simulink library "scp"  (R2021b)
settings: Solver=VariableStepAuto  StartTime=0.0  StopTime=10.0  RelTol=1e-3
libraries: FVT_lib x1
settings Model: Creator=FVT23118  LastModifiedBy=FVT23010

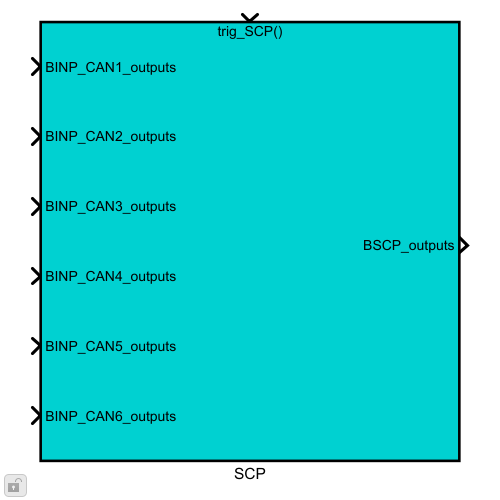
[thumbnail: Simulink's stored preview of the top-level diagram]
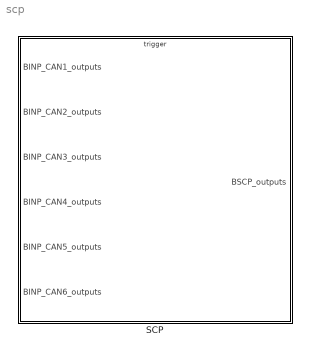
== system scp ==
  SCP : Subsystem

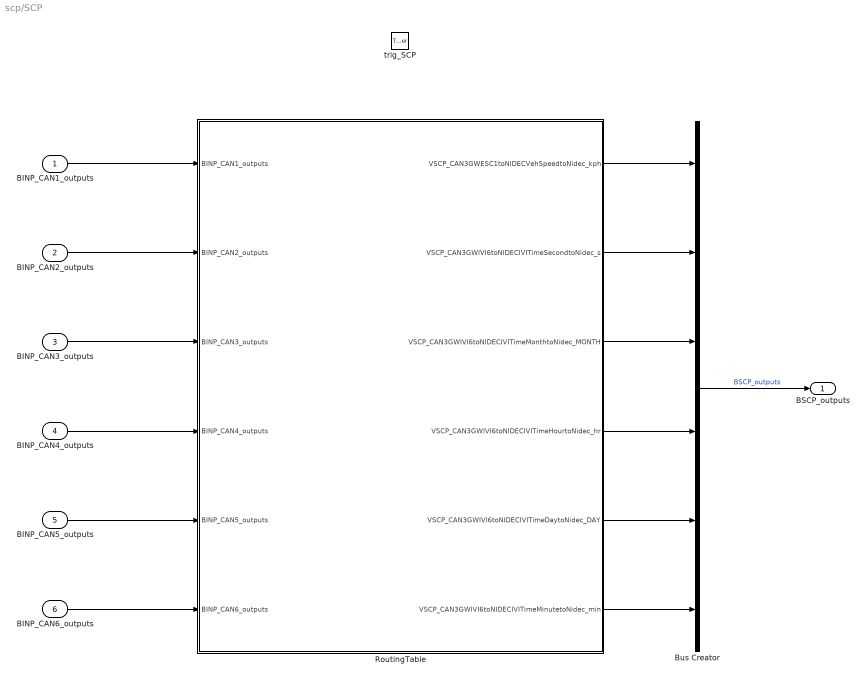
== system scp/SCP ==
  BINP_CAN1_outputs : Inport  OutDataTypeStr=Bus: BINP_CAN1_outputs
  BINP_CAN2_outputs : Inport  Port=2  OutDataTypeStr=Bus: BINP_CAN2_outputs
  BINP_CAN3_outputs : Inport  Port=3  OutDataTypeStr=Bus: BINP_CAN3_outputs
  BINP_CAN4_outputs : Inport  Port=4  OutDataTypeStr=Bus: BINP_CAN4_outputs
  BINP_CAN5_outputs : Inport  Port=5  OutDataTypeStr=Bus: BINP_CAN5_outputs
  BINP_CAN6_outputs : Inport  Port=6  OutDataTypeStr=Bus: BINP_CAN6_outputs
  trig_SCP : TriggerPort  TriggerType=function-call  VariantControl=(inherit)  PortDimensions=1
  Bus Creator : BusCreator  Inputs=6
  RoutingTable : Subsystem
  BSCP_outputs : Outport  OutDataTypeStr=Bus: BSCP_outputs
  wires:
  Bus Creator/1 -> BSCP_outputs/1  "BSCP_outputs"
  BINP_CAN1_outputs/1 -> RoutingTable/1(BINP_CAN1_outputs)
  BINP_CAN4_outputs/1 -> RoutingTable/4(BINP_CAN4_outputs)
  BINP_CAN3_outputs/1 -> RoutingTable/3(BINP_CAN3_outputs)
  BINP_CAN2_outputs/1 -> RoutingTable/2(BINP_CAN2_outputs)
  BINP_CAN5_outputs/1 -> RoutingTable/5(BINP_CAN5_outputs)
  BINP_CAN6_outputs/1 -> RoutingTable/6(BINP_CAN6_outputs)
  RoutingTable/1("VSCP_CAN3GWESC1toNIDECVehSpeedtoNidec_kph ") -> Bus Creator/1
  RoutingTable/2(VSCP_CAN3GWIVI6toNIDECIVITimeSecondtoNidec_s) -> Bus Creator/2
  RoutingTable/3(VSCP_CAN3GWIVI6toNIDECIVITimeMonthtoNidec_MONTH) -> Bus Creator/3
  RoutingTable/4(VSCP_CAN3GWIVI6toNIDECIVITimeHourtoNidec_hr) -> Bus Creator/4
  RoutingTable/5(VSCP_CAN3GWIVI6toNIDECIVITimeDaytoNidec_DAY) -> Bus Creator/5
  RoutingTable/6(VSCP_CAN3GWIVI6toNIDECIVITimeMinutetoNidec_min) -> Bus Creator/6

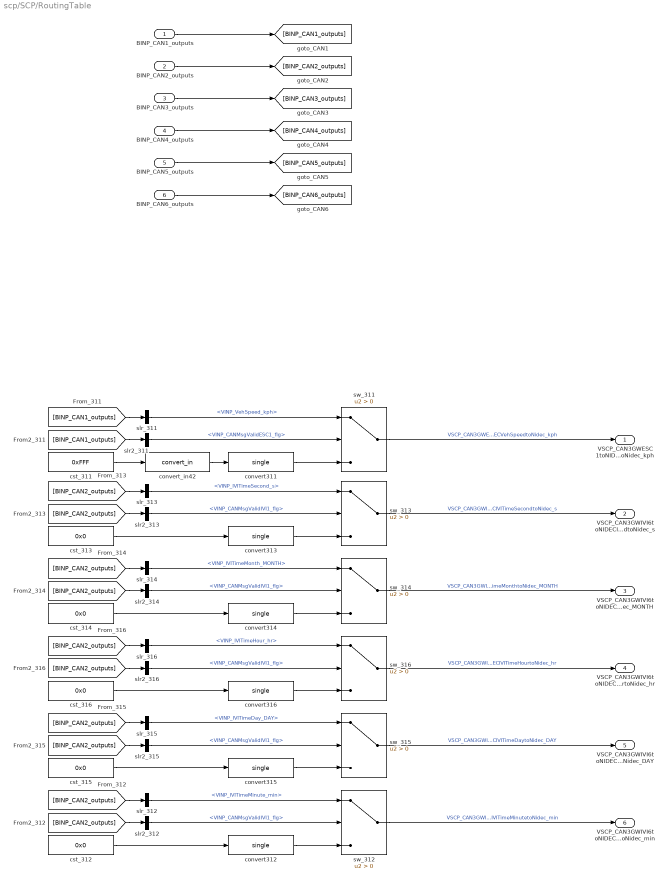
== system scp/SCP/RoutingTable ==
  BINP_CAN1_outputs : Inport
  BINP_CAN2_outputs : Inport  Port=2
  BINP_CAN3_outputs : Inport  Port=3
  BINP_CAN4_outputs : Inport  Port=4
  BINP_CAN5_outputs : Inport  Port=5
  BINP_CAN6_outputs : Inport  Port=6
  convert{311..316} (6 alike) : DataTypeConversion  OutDataTypeStr=single
  convert_in42 : FVT_lib/hal/convert_in  gain=0.125  offset=0
  cst_311 : Constant  Value=0xFFF
  cst_{312..316} (5 alike) : Constant  Value=0x0
  slr2_311 : BusSelector  OutputSignals=VINP_CANMsgValidESC1_flg
  slr2_{312..316} (5 alike) : BusSelector  OutputSignals=VINP_CANMsgValidIVI1_flg
  slr_311 : BusSelector  OutputSignals=VINP_VehSpeed_kph
  slr_312 : BusSelector  OutputSignals=VINP_IVITimeMinute_min
  slr_313 : BusSelector  OutputSignals=VINP_IVITimeSecond_s
  slr_314 : BusSelector  OutputSignals=VINP_IVITimeMonth_MONTH
  slr_315 : BusSelector  OutputSignals=VINP_IVITimeDay_DAY
  slr_316 : BusSelector  OutputSignals=VINP_IVITimeHour_hr
  sw_{311..316} (6 alike) : Switch  Criteria=u2 > Threshold
  "VSCP_CAN3GWESC1toNIDECVehSpeedtoNidec_kph " : Outport
  VSCP_CAN3GWIVI6toNIDECIVITimeSecondtoNidec_s : Outport  Port=2
  VSCP_CAN3GWIVI6toNIDECIVITimeMonthtoNidec_MONTH : Outport  Port=3
  VSCP_CAN3GWIVI6toNIDECIVITimeHourtoNidec_hr : Outport  Port=4
  VSCP_CAN3GWIVI6toNIDECIVITimeDaytoNidec_DAY : Outport  Port=5
  VSCP_CAN3GWIVI6toNIDECIVITimeMinutetoNidec_min : Outport  Port=6
  wires:
  BINP_CAN1_outputs/1 -> [BINP_CAN1_outputs]
  BINP_CAN2_outputs/1 -> [BINP_CAN2_outputs]
  BINP_CAN3_outputs/1 -> [BINP_CAN3_outputs]
  BINP_CAN4_outputs/1 -> [BINP_CAN4_outputs]
  BINP_CAN5_outputs/1 -> [BINP_CAN5_outputs]
  BINP_CAN6_outputs/1 -> [BINP_CAN6_outputs]
  convert315/1 -> sw_315/3
  sw_314/1 -> VSCP_CAN3GWIVI6toNIDECIVITimeMonthtoNidec_MONTH/1  "VSCP_CAN3GWIVI6toNIDECIVITimeMonthtoNidec_MONTH"
  [BINP_CAN2_outputs] -> slr_316/1
  [BINP_CAN1_outputs] -> slr2_311/1
  [BINP_CAN2_outputs] -> slr_313/1
  [BINP_CAN1_outputs] -> slr_311/1
  sw_313/1 -> VSCP_CAN3GWIVI6toNIDECIVITimeSecondtoNidec_s/1  "VSCP_CAN3GWIVI6toNIDECIVITimeSecondtoNidec_s"
  slr_316/1 -> sw_316/1  "<VINP_IVITimeHour_hr>"
  sw_315/1 -> VSCP_CAN3GWIVI6toNIDECIVITimeDaytoNidec_DAY/1  "VSCP_CAN3GWIVI6toNIDECIVITimeDaytoNidec_DAY"
  convert311/1 -> sw_311/3
  [BINP_CAN2_outputs] -> slr2_312/1
  [BINP_CAN2_outputs] -> slr2_313/1
  slr_313/1 -> sw_313/1  "<VINP_IVITimeSecond_s>"
  slr2_313/1 -> sw_313/2  "<VINP_CANMsgValidIVI1_flg>"
  slr2_315/1 -> sw_315/2  "<VINP_CANMsgValidIVI1_flg>"
  slr_312/1 -> sw_312/1  "<VINP_IVITimeMinute_min>"
  [BINP_CAN2_outputs] -> slr_312/1
  convert_in42/1 -> convert311/1
  slr2_312/1 -> sw_312/2  "<VINP_CANMsgValidIVI1_flg>"
  slr2_314/1 -> sw_314/2  "<VINP_CANMsgValidIVI1_flg>"
  cst_315/1 -> convert315/1
  [BINP_CAN2_outputs] -> slr_314/1
  sw_316/1 -> VSCP_CAN3GWIVI6toNIDECIVITimeHourtoNidec_hr/1  "VSCP_CAN3GWIVI6toNIDECIVITimeHourtoNidec_hr"
  sw_311/1 -> "VSCP_CAN3GWESC1toNIDECVehSpeedtoNidec_kph "/1  "VSCP_CAN3GWESC1toNIDECVehSpeedtoNidec_kph"
  cst_314/1 -> convert314/1
  convert314/1 -> sw_314/3
  slr_315/1 -> sw_315/1  "<VINP_IVITimeDay_DAY>"
  convert312/1 -> sw_312/3
  [BINP_CAN2_outputs] -> slr_315/1
  sw_312/1 -> VSCP_CAN3GWIVI6toNIDECIVITimeMinutetoNidec_min/1  "VSCP_CAN3GWIVI6toNIDECIVITimeMinutetoNidec_min"
  cst_316/1 -> convert316/1
  slr2_311/1 -> sw_311/2  "<VINP_CANMsgValidESC1_flg>"
  convert316/1 -> sw_316/3
  [BINP_CAN2_outputs] -> slr2_314/1
  cst_311/1 -> convert_in42/1
  [BINP_CAN2_outputs] -> slr2_315/1
  slr_314/1 -> sw_314/1  "<VINP_IVITimeMonth_MONTH>"
  convert313/1 -> sw_313/3
  slr_311/1 -> sw_311/1  "<VINP_VehSpeed_kph>"
  slr2_316/1 -> sw_316/2  "<VINP_CANMsgValidIVI1_flg>"
  cst_312/1 -> convert312/1
  [BINP_CAN2_outputs] -> slr2_316/1
  cst_313/1 -> convert313/1
